simulink model "simucarr"  (R2024b)
settings: Solver=VariableStepAuto  StartTime=0.0  StopTime=10.0  RelTol=1e-3
InitFcn:
  | m1=290;
  | b1=1000;
  | m2=59;
  | k1=16182;
  | f=0;
  | k2=19000;
  | z1 =0.05;
  | z2 =0;
settings Model: Creator=sanch  LastModifiedBy=sanch

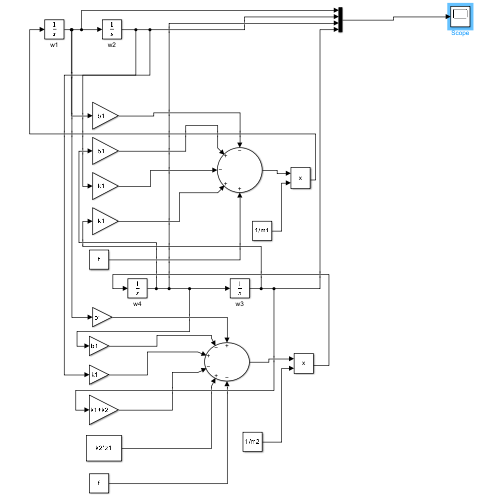
[thumbnail: Simulink's stored preview of the top-level diagram]
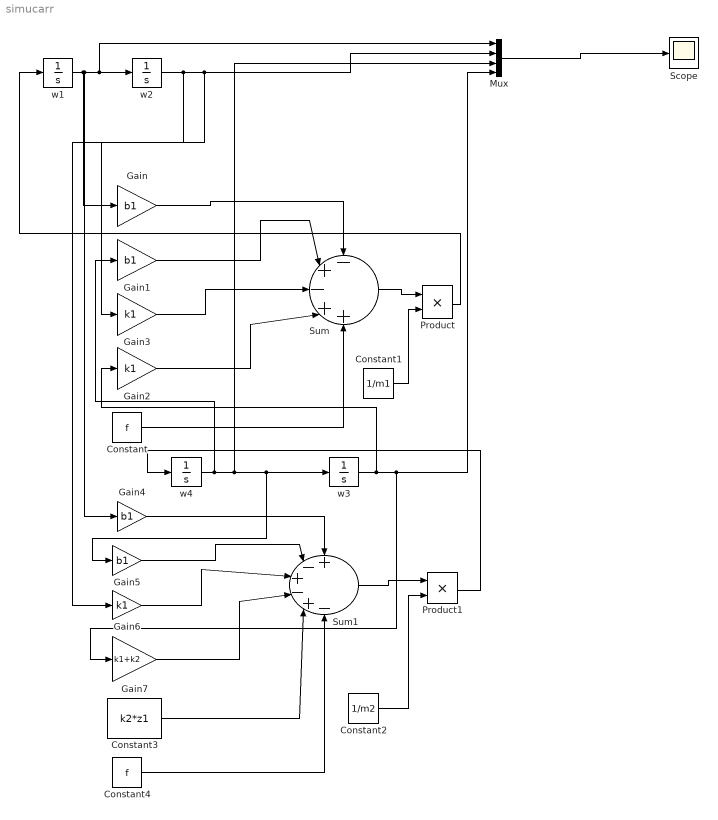
== system simucarr ==
  Constant : Constant  Value=f
  Constant1 : Constant  Value=1/m1
  Constant2 : Constant  Value=1/m2
  Constant3 : Constant  Value=k2*z1
  Constant4 : Constant  Value=f
  Gain{,1,4..5} (4 alike) : Gain  Gain=b1
  Gain2 : Gain  Gain=k1
  Gain3 : Gain  Gain=k1
  Gain6 : Gain  Gain=k1
  Gain7 : Gain  Gain=k1+k2
  Mux : Mux
  Product : Product
  Product1 : Product
  Scope : Scope
  Sum : Sum  Inputs=-+-++
  Sum1 : Sum  Inputs=+-+-+-
  w{1..4} (4 alike) : Integrator
  wires:
  Gain/1 -> Sum/1
  Gain1/1 -> Sum/2
  Gain3/1 -> Sum/3
  Gain2/1 -> Sum/4
  Mux/1 -> Scope/1
  Constant/1 -> Sum/5
  Sum/1 -> Product/1
  Constant1/1 -> Product/2
  Gain7/1 -> Sum1/4
  Gain6/1 -> Sum1/3
  Gain5/1 -> Sum1/2
  Gain4/1 -> Sum1/1
  Sum1/1 -> Product1/1
  Constant2/1 -> Product1/2
  Product1/1 -> w4/1
  w4/1 -> Gain1/1, Mux/3, Gain5/1, w3/1
  w3/1 -> Gain2/1, Gain7/1, Mux/4
  w1/1 -> Gain/1, w2/1, Mux/1, Gain4/1
  w2/1 -> Gain3/1, Gain6/1, Mux/2
  Product/1 -> w1/1
  Constant3/1 -> Sum1/5
  Constant4/1 -> Sum1/6
